simulink model "core_logic"  (R2024b)
settings: Solver=FixedStepAuto  StartTime=0.0  StopTime=1000  FixedStep=10e-3  RelTol=1e-3
libraries: SignalEditorBlockLib x2
settings Model: SimulationMode=accelerator  Creator=Nitesh  LastModifiedBy=Nitesh

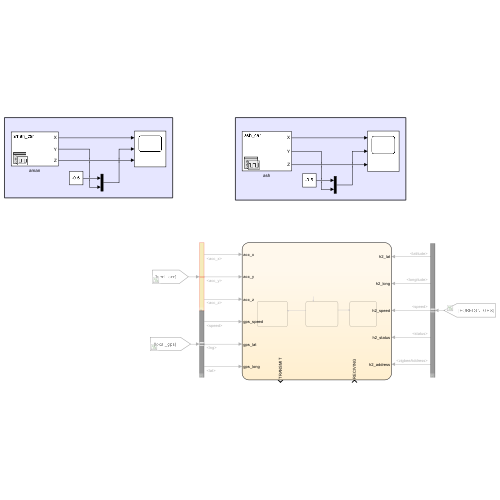
[thumbnail: Simulink's stored preview of the top-level diagram]
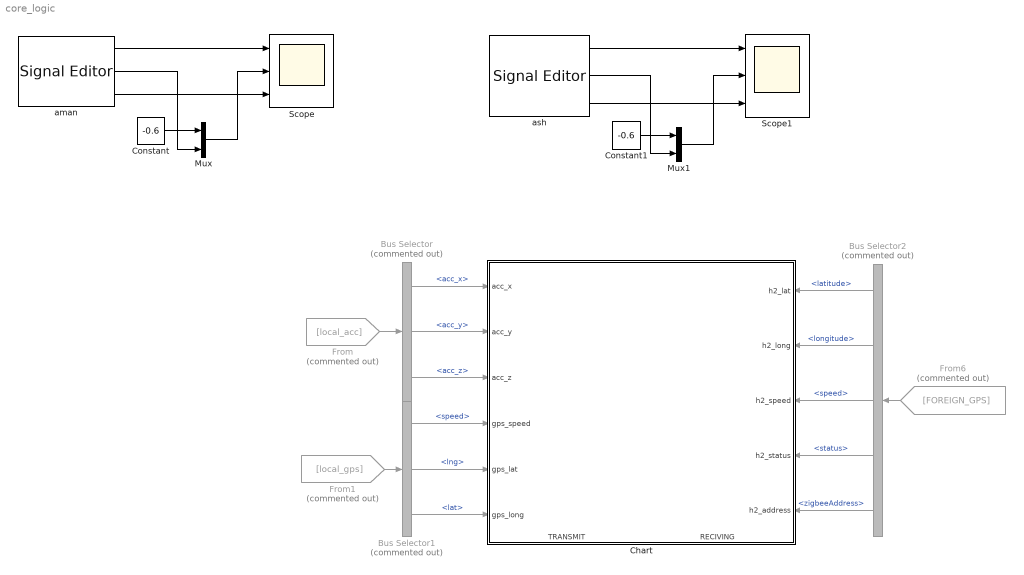
== system core_logic ==
  Bus Selector : BusSelector  Commented=on  OutputSignals=acc_x,acc_y,acc_z
  Bus Selector1 : BusSelector  Commented=on  OutputSignals=speed,lng,lat
  Bus Selector2 : BusSelector  Commented=on  OutputSignals=latitude,longitude,speed,status,zigbeeAddress
  Chart : Stateflow chart  TreatAsAtomicUnit=on
      settings: PortSchema="{\"entries\":[{\"content\":{\"sides\":[{\"content\":{\"connectorIds\":[\"In1\",\"In2\",\"In3\",\"In6\",\"In4\",\"In5\"]},\"type\":\"ConnectorPlacement.EquallySpacedRectSide\",\"uuid\":\"ee7c9145-97fe-42bf-b38f-25095debb339\"},{\"content\":{\"connectorIds\":[\"In8\",\"In9\",\"In10\",\"In11\",\"In12\"],\"side\":\"RIGHT\"},\"type\":\"ConnectorPlacement.EquallySpacedRectSide\",\"uuid\":\"6ad3cc48-74a8-47e1-8b84-b3331846d199\"},{\"content\":{\"side\":\"TOP\"},\"type\":\"ConnectorPlacement.EquallySpacedRectSide\",\"uuid\":\"0e80e778-40c2-414e-b172-27c343627a22\"},{\"content\":{\"connectorIds\":[\"Out1\",\"In7\"],\"side\":\"BOTTOM\"},\"type\":\"ConnectorPlacement.EquallySpacedRectSide\",\"uuid\":\"8c076511-fb77-4abd-9a6c-f32e2686fd08\"}]},\"type\":\"ConnectorPlacement.EquallySpacedConnector\",\"uuid\":\"44f6d062-1c8f-4774-b93e-5476bfb914ed\"}],\"packageUris\":[\"http://schema.mathworks.com/mf0/Connector/R2020b\"],\"version\":\"1.0\"}"
  Constant : Constant  Value=-0.6
  Constant1 : Constant  Value=-0.6
  From : From  Commented=on  GotoTag=local_acc
  From1 : From  Commented=on  GotoTag=local_gps
  From6 : From  Commented=on  GotoTag=FOREIGN_GPS
  Mux : Mux  Inputs=2
  Mux1 : Mux  Inputs=2
  Scope : Scope  NumInputPorts=3
  Scope1 : Scope  NumInputPorts=3
  aman : SignalEditorBlockLib/Signal Editor  FileName=acc_data.mat  ActiveScenario=aman_car  ActiveSignal=X  IsBus=off  OutputBusObjectStr=Bus: BusObject  SampleTime=0  ZeroCross=off  OutputAfterFinalValue=Setting to zero  Unit=inherit  PreserveSignalName=on  ApplySigPropsToAllScenarios=on  ApplySigPropsToAllSignals=on
  ash : SignalEditorBlockLib/Signal Editor  FileName=acc_data.mat  ActiveScenario=ash_car  ActiveSignal=X  IsBus=off  OutputBusObjectStr=Bus: BusObject  SampleTime=0  ZeroCross=off  OutputAfterFinalValue=Setting to zero  Unit=inherit  PreserveSignalName=on  ApplySigPropsToAllScenarios=on  ApplySigPropsToAllSignals=off
  wires:
  aman/1 -> Scope/1
  aman/2 -> Mux/2
  aman/3 -> Scope/3
  ash/1 -> Scope1/1
  ash/3 -> Scope1/3
  Constant/1 -> Mux/1
  Mux/1 -> Scope/2
  Mux1/1 -> Scope1/2
  Constant1/1 -> Mux1/1
  ash/2 -> Mux1/2
  Bus Selector1/3 -> Chart/5(gps_long)  "<lat>"
  Bus Selector/3 -> Chart/3(acc_z)  "<acc_z>"
  Bus Selector2/5 -> Chart/12(h2_address)  "<zigbeeAddress>"
  Bus Selector/1 -> Chart/1(acc_x)  "<acc_x>"
  Bus Selector2/2 -> Chart/9(h2_long)  "<longitude>"
  From1/1 -> Bus Selector1/1
  From/1 -> Bus Selector/1
  Bus Selector2/4 -> Chart/11(h2_status)  "<status>"
  Bus Selector1/2 -> Chart/4(gps_lat)  "<lng>"
  Bus Selector2/3 -> Chart/10(h2_speed)  "<speed>"
  Bus Selector/2 -> Chart/2(acc_y)  "<acc_y>"
  From6/1 -> Bus Selector2/1
  Bus Selector1/1 -> Chart/6(gps_speed)  "<speed>"
  Bus Selector2/1 -> Chart/8(h2_lat)  "<latitude>"

== stateflow chart core_logic/Chart ==
  state nearby_crash
  state normal
    entry:
    TRANSMIT=false
  state crashed
    entry:
    TRANSMIT=true
  (default) -> normal
  normal -> crashed [order 2] : [acc_y<-0.6]
  normal -> nearby_crash [order 1] : [RECIVING==true]
  data: TRANSMIT output boolean; acc_x input; acc_y input; acc_z input; gps_lat input; gps_long input; gps_speed input; RECIVING input boolean; h2_lat input; h2_long input; h2_speed input; h2_status input; h2_address input
  events: sudden_breaking local FUNCTION_CALL_EVENT
